simulink model "testModel"  (R2019b)
settings: Solver=FixedStepAuto  StartTime=0.0  StopTime=10  FixedStep=.001  RelTol=1e-3
undefined symbols (not defined in the file or in its folder): DiscIntNeverNeededParam
libraries: simulink x3
settings Model: Creator=Nick  LastModifiedBy=Nick

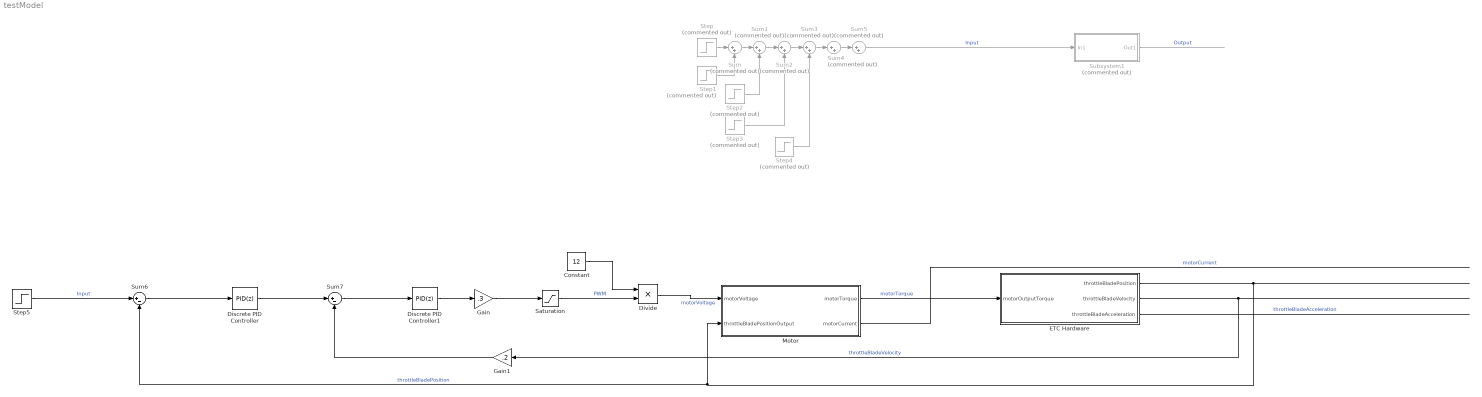
== system testModel ==
  Constant : Constant  Value=12
  Discrete PID Controller : simulink/Continuous/PID Controller  Controller=PID  Form=Parallel  TimeDomain=Discrete-time  SampleTime=-1  IntegratorMethod=Forward Euler  FilterMethod=Forward Euler  ControllerParametersSource=internal  P=10  I=0  D=0  UseFilter=on  N=100  TunerSelectOption=Transfer Function Based (PID Tuner App)  InitialConditionSource=internal  InitialConditionForIntegrator=0  InitialConditionForFilter=0  DifferentiatorICPrevScaledInput=0  ExternalReset=none  TrackingMode=off  Kt=1  LimitOutput=off  UpperSaturationLimit=inf  LowerSaturationLimit=-inf  LinearizeAsGain=off  AntiWindupMode=none  Kb=1  POutMin=[]  POutMax=[]  IOutMin=[]  IOutMax=[]  DOutMin=[]  DOutMax=[]  NOutMin=[]  NOutMax=[]  SumOutMin=[]  SumOutMax=[]  SaturationOutMin=[]  SaturationOutMax=[]  PParamMin=[]  PParamMax=[]  IParamMin=[]  IParamMax=[]  DParamMin=[]  DParamMax=[]  NParamMin=[]  NParamMax=[]  KbParamMin=[]  KbParamMax=[]  KtParamMin=[]  KtParamMax=[]  KbOutMin=[]  KbOutMax=[]  KtOutMin=[]  KtOutMax=[]  IntegratorOutMin=[]  IntegratorOutMax=[]  FilterOutMin=[]  FilterOutMax=[]  SumI1OutMin=[]  SumI1OutMax=[]  SumI2OutMin=[]  SumI2OutMax=[]  SumI3OutMin=[]  SumI3OutMax=[]  SumI4OutMin=[]  SumI4OutMax=[]  SumDOutMin=[]  SumDOutMax=[]  DifferentiatorOutMin=[]  DifferentiatorOutMax=[]  FilterDiffOutCoefMin=[]  FilterDiffOutCoefMax=[]  ReciprocalOutMin=[]  ReciprocalOutMax=[]  SumDenOutMin=[]  SumDenOutMax=[]  SumNumOutMin=[]  SumNumOutMax=[]  DivideOutMin=[]  DivideOutMax=[]  IntegratorContinuousStateAttributes=''  IntegratorStateMustResolveToSignalObject=off  IntegratorRTWStateStorageClass=Auto  FilterContinuousStateAttributes=''  FilterStateMustResolveToSignalObject=off  FilterRTWStateStorageClass=Auto  ParallelPVariant=InternalParameters  IdealPVariant=Disabled  IVariant=InternalParameters  DVariant=InternalParameters  IntegratorVariant=Discrete  SatVariant=Disabled  AWVariant=Passthrough  PCopyVariant=Disabled  TRVariant=Disabled  FdbkBlocksVariant=Forward  IdealPFdbkVariant=Disabled  SatFdbkVariant=Disabled  DerivativeFilterVariant=ForwardEulerFilter  NVariant=InternalParameters  NCopyVariant=Disabled  FilterICVariant=InternalICsFilter  IntegratorICVariant=InternalICs  ExternalResetVariant=Disabled  TRSumVariant=Passthrough  SumFdbkVariant=Disabled  SumVariant=Sum_PID
  Discrete PID Controller1 : simulink/Continuous/PID Controller  Controller=PID  Form=Parallel  TimeDomain=Discrete-time  SampleTime=-1  IntegratorMethod=Forward Euler  FilterMethod=Forward Euler  ControllerParametersSource=internal  P=1  I=2  D=0  UseFilter=on  N=100  TunerSelectOption=Transfer Function Based (PID Tuner App)  InitialConditionSource=internal  InitialConditionForIntegrator=0  InitialConditionForFilter=0  DifferentiatorICPrevScaledInput=0  ExternalReset=none  TrackingMode=off  Kt=1  LimitOutput=off  UpperSaturationLimit=inf  LowerSaturationLimit=-inf  LinearizeAsGain=off  AntiWindupMode=none  Kb=1  POutMin=[]  POutMax=[]  IOutMin=[]  IOutMax=[]  DOutMin=[]  DOutMax=[]  NOutMin=[]  NOutMax=[]  SumOutMin=[]  SumOutMax=[]  SaturationOutMin=[]  SaturationOutMax=[]  PParamMin=[]  PParamMax=[]  IParamMin=[]  IParamMax=[]  DParamMin=[]  DParamMax=[]  NParamMin=[]  NParamMax=[]  KbParamMin=[]  KbParamMax=[]  KtParamMin=[]  KtParamMax=[]  KbOutMin=[]  KbOutMax=[]  KtOutMin=[]  KtOutMax=[]  IntegratorOutMin=[]  IntegratorOutMax=[]  FilterOutMin=[]  FilterOutMax=[]  SumI1OutMin=[]  SumI1OutMax=[]  SumI2OutMin=[]  SumI2OutMax=[]  SumI3OutMin=[]  SumI3OutMax=[]  SumI4OutMin=[]  SumI4OutMax=[]  SumDOutMin=[]  SumDOutMax=[]  DifferentiatorOutMin=[]  DifferentiatorOutMax=[]  FilterDiffOutCoefMin=[]  FilterDiffOutCoefMax=[]  ReciprocalOutMin=[]  ReciprocalOutMax=[]  SumDenOutMin=[]  SumDenOutMax=[]  SumNumOutMin=[]  SumNumOutMax=[]  DivideOutMin=[]  DivideOutMax=[]  IntegratorContinuousStateAttributes=''  IntegratorStateMustResolveToSignalObject=off  IntegratorRTWStateStorageClass=Auto  FilterContinuousStateAttributes=''  FilterStateMustResolveToSignalObject=off  FilterRTWStateStorageClass=Auto  ParallelPVariant=InternalParameters  IdealPVariant=Disabled  IVariant=InternalParameters  DVariant=InternalParameters  IntegratorVariant=Discrete  SatVariant=Disabled  AWVariant=Passthrough  PCopyVariant=Disabled  TRVariant=Disabled  FdbkBlocksVariant=Forward  IdealPFdbkVariant=Disabled  SatFdbkVariant=Disabled  DerivativeFilterVariant=ForwardEulerFilter  NVariant=InternalParameters  NCopyVariant=Disabled  FilterICVariant=InternalICsFilter  IntegratorICVariant=InternalICs  ExternalResetVariant=Disabled  TRSumVariant=Passthrough  SumFdbkVariant=Disabled  SumVariant=Sum_PID
  Divide : Product  Inputs=**
  ETC Hardware : Subsystem
  Gain : Gain  Gain=.3
  Gain1 : Gain  Gain=.2
  Motor : Subsystem
  Saturation : Saturate  UpperLimit=.5  LowerLimit=0
  Step : Step  Commented=on  SampleTime=0
  Step1 : Step  Commented=on  Time=2  After=-1  SampleTime=0
  Step2 : Step  Commented=on  Time=3  After=2  SampleTime=0
  Step3 : Step  Commented=on  Time=4  After=-2  SampleTime=0
  Step4 : Step  Commented=on  Time=5  After=5  SampleTime=0
  Step5 : Step  SampleTime=0
  Subsystem1 : Subsystem  Commented=on
  Sum{,1..5} (6 alike) : Sum  Commented=on  Inputs=|++
  Sum6 : Sum  Inputs=|+-
  Sum7 : Sum  Inputs=|+-
  wires:
  Subsystem1/1(Out1) -> ?  "Output"
  Sum5/1 -> Subsystem1/1(In1)  "Input"
  Step/1 -> Sum/1
  Sum/1 -> Sum1/1
  Sum1/1 -> Sum2/1
  Sum2/1 -> Sum3/1
  Sum3/1 -> Sum4/1
  Sum4/1 -> Sum5/1
  Step1/1 -> Sum/2
  Step2/1 -> Sum1/2
  Step3/1 -> Sum2/2
  Step4/1 -> Sum3/2
  ETC Hardware/2(throttleBladeVelocity) -> Gain1/1  "throttleBladeVelocity"
  Gain/1 -> Saturation/1
  ETC Hardware/3(throttleBladeAcceleration) -> ?  "throttleBladeAcceleration"
  Motor/1(motorTorque) -> ETC Hardware/1(motorOutputTorque)  "motorTorque"
  Motor/2(motorCurrent) -> ?  "motorCurrent"
  ETC Hardware/1(throttleBladePosition) -> Sum6/2, Motor/2(throttleBladePositionOutput)  "throttleBladePosition"
  Sum6/1 -> Discrete PID Controller/1
  Sum7/1 -> Discrete PID Controller1/1
  Discrete PID Controller/1 -> Sum7/1
  Discrete PID Controller1/1 -> Gain/1
  Step5/1 -> Sum6/1  "Input"
  Divide/1 -> Motor/1(motorVoltage)  "motorVoltage"
  Saturation/1 -> Divide/2  "PWM"
  Constant/1 -> Divide/1
  Gain1/1 -> Sum7/2

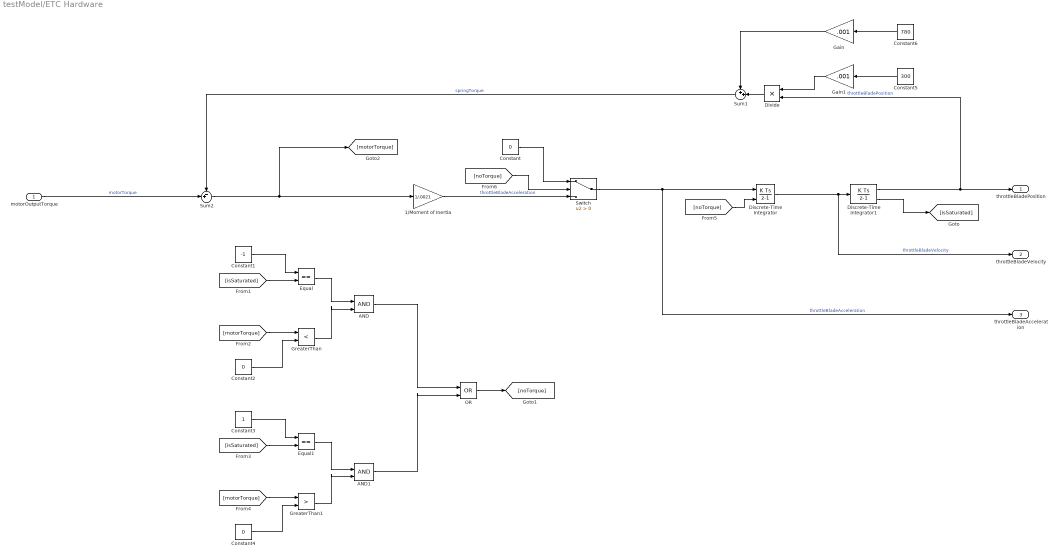
== system testModel/ETC Hardware ==
  motorOutputTorque : Inport
  1/Moment of Inertia : Gain  Gain=1/.0021
  AND : Logic  IconShape=distinctive  AllPortsSameDT=off  OutDataTypeStr=boolean
  AND1 : Logic  IconShape=distinctive  AllPortsSameDT=off  OutDataTypeStr=boolean
  Constant : Constant  Value=0
  Constant1 : Constant  Value=-1
  Constant2 : Constant  Value=0
  Constant3 : Constant
  Constant4 : Constant  Value=0
  Constant5 : Constant  Value=300
  Constant6 : Constant  Value=780
  Discrete-Time Integrator : DiscreteIntegrator  ExternalReset=level  SampleTime=-1  ICPrevOutput=DiscIntNeverNeededParam  ICPrevScaledInput=DiscIntNeverNeededParam
  Discrete-Time Integrator1 : DiscreteIntegrator  SampleTime=-1  LimitOutput=on  UpperSaturationLimit=1.5708  LowerSaturationLimit=0  ShowSaturationPort=on  ICPrevOutput=DiscIntNeverNeededParam  ICPrevScaledInput=DiscIntNeverNeededParam
  Divide : Product  Inputs=**
  Equal : RelationalOperator  Operator===  OutDataTypeStr=boolean  RndMeth=Simplest
  Equal1 : RelationalOperator  Operator===  OutDataTypeStr=boolean  RndMeth=Simplest
  Gain : Gain  Gain=.001
  Gain1 : Gain  Gain=.001
  GreaterThan : RelationalOperator  Operator=<  OutDataTypeStr=boolean  RndMeth=Simplest
  GreaterThan1 : RelationalOperator  Operator=>  OutDataTypeStr=boolean  RndMeth=Simplest
  OR : Logic  Operator=OR  IconShape=distinctive  AllPortsSameDT=off  OutDataTypeStr=boolean
  Sum1 : Sum  Inputs=++|
  Sum2 : Sum  Inputs=-+|
  Switch : Switch  Criteria=u2 > Threshold
  throttleBladePosition : Outport
  throttleBladeVelocity : Outport  Port=2
  throttleBladeAcceleration : Outport  Port=3
  wires:
  Constant5/1 -> Gain1/1
  Gain1/1 -> Divide/1
  Constant6/1 -> Gain/1
  motorOutputTorque/1 -> Sum2/2  "motorTorque"
  Sum1/1 -> Sum2/1  "springTorque"
  Switch/1 -> Discrete-Time Integrator/1, throttleBladeAcceleration/1  "throttleBladeAcceleration"
  Discrete-Time Integrator/1 -> throttleBladeVelocity/1, Discrete-Time Integrator1/1  "throttleBladeVelocity"
  Discrete-Time Integrator1/1 -> throttleBladePosition/1, Divide/2  "throttleBladePosition"
  Divide/1 -> Sum1/2
  Gain/1 -> Sum1/1
  Sum2/1 -> 1/Moment of Inertia/1, [motorTorque]
  Constant1/1 -> Equal/1
  Equal/1 -> AND/1
  Discrete-Time Integrator1/2 -> [isSaturated]
  OR/1 -> [noTorque]
  [isSaturated] -> Equal/2
  GreaterThan/1 -> AND/2
  Constant2/1 -> GreaterThan/2
  [motorTorque] -> GreaterThan/1
  [motorTorque] -> GreaterThan1/1
  Constant4/1 -> GreaterThan1/2
  [isSaturated] -> Equal1/2
  Constant3/1 -> Equal1/1
  Equal1/1 -> AND1/1
  GreaterThan1/1 -> AND1/2
  AND/1 -> OR/1
  AND1/1 -> OR/2
  [noTorque] -> Discrete-Time Integrator/2
  1/Moment of Inertia/1 -> Switch/3  "throttleBladeAcceleration"
  [noTorque] -> Switch/2
  Constant/1 -> Switch/1

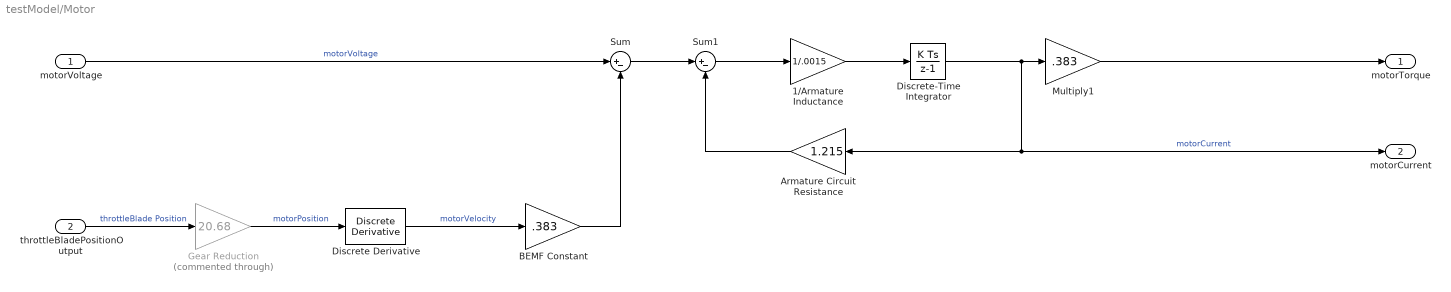
== system testModel/Motor ==
  motorVoltage : Inport
  throttleBladePositionOutput : Inport  Port=2
  1/Armature Inductance : Gain  Gain=1/.0015
  Armature Circuit Resistance : Gain  Gain=1.215
  BEMF Constant : Gain  Gain=.383
  Discrete Derivative : simulink/Discrete/Discrete Derivative  gainval=1.0  ICPrevScaledInput=0.0  OutMin=[]  OutMax=[]  OutDataType=fixdt(1, 16)  OutScaling=2^-10  DoSatur=off
  Discrete-Time Integrator : DiscreteIntegrator  SampleTime=-1  ICPrevOutput=DiscIntNeverNeededParam  ICPrevScaledInput=DiscIntNeverNeededParam
  Gear Reduction : Gain  Commented=through  Gain=20.68
  Multiply1 : Gain  Gain=.383
  Sum : Sum  Inputs=|+-
  Sum1 : Sum  Inputs=|+-
  motorTorque : Outport
  motorCurrent : Outport  Port=2
  wires:
  Discrete-Time Integrator/1 -> Armature Circuit Resistance/1, motorCurrent/1, Multiply1/1  "motorCurrent"
  Multiply1/1 -> motorTorque/1
  motorVoltage/1 -> Sum/1  "motorVoltage"
  Armature Circuit Resistance/1 -> Sum1/2
  Sum1/1 -> 1/Armature Inductance/1
  1/Armature Inductance/1 -> Discrete-Time Integrator/1
  Sum/1 -> Sum1/1
  BEMF Constant/1 -> Sum/2
  throttleBladePositionOutput/1 -> Gear Reduction/1  "throttleBlade Position"
  Gear Reduction/1 -> Discrete Derivative/1  "motorPosition"
  Discrete Derivative/1 -> BEMF Constant/1  "motorVelocity"

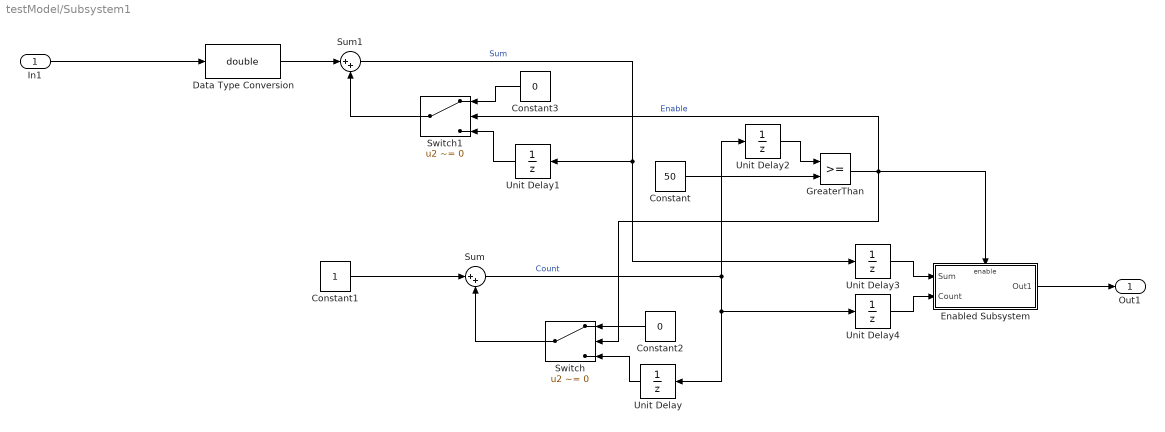
== system testModel/Subsystem1 ==
  In1 : Inport
  Constant : Constant  Value=50
  Constant1 : Constant
  Constant2 : Constant  Value=0
  Constant3 : Constant  Value=0
  Data Type Conversion : DataTypeConversion  OutDataTypeStr=double
  Enabled Subsystem : Subsystem  TreatAsAtomicUnit=on
  GreaterThan : RelationalOperator  OutDataTypeStr=boolean  RndMeth=Simplest
  Sum : Sum  Inputs=|++
  Sum1 : Sum  Inputs=|++
  Switch : Switch  Criteria=u2 ~= 0  Threshold=50
  Switch1 : Switch  Criteria=u2 ~= 0  Threshold=50
  Unit Delay{,1..4} (5 alike) : UnitDelay  SampleTime=-1  HasFrameUpgradeWarning=on
  Out1 : Outport
  wires:
  In1/1 -> Data Type Conversion/1
  Enabled Subsystem/1(Out1) -> Out1/1
  Constant/1 -> GreaterThan/2
  Sum1/1 -> Unit Delay3/1, Unit Delay1/1  "Sum"
  Sum/1 -> Unit Delay4/1, Unit Delay/1, Unit Delay2/1  "Count"
  GreaterThan/1 -> Switch1/2, Switch/2, Enabled Subsystem/Enable  "Enable"
  Constant1/1 -> Sum/1
  Unit Delay/1 -> Switch/3
  Constant2/1 -> Switch/1
  Switch/1 -> Sum/2
  Data Type Conversion/1 -> Sum1/1
  Unit Delay1/1 -> Switch1/3
  Constant3/1 -> Switch1/1
  Switch1/1 -> Sum1/2
  Unit Delay2/1 -> GreaterThan/1
  Unit Delay4/1 -> Enabled Subsystem/2(Count)
  Unit Delay3/1 -> Enabled Subsystem/1(Sum)

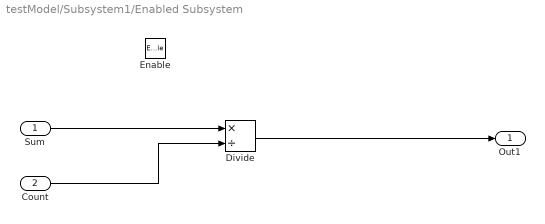
== system testModel/Subsystem1/Enabled Subsystem ==
  Sum : Inport
  Count : Inport  Port=2
  Enable : EnablePort
  Divide : Product  Inputs=*/
  Out1 : Outport
  wires:
  Sum/1 -> Divide/1
  Count/1 -> Divide/2
  Divide/1 -> Out1/1
